simulink model "s0418"  (Simulink 7.0)
settings: Solver=ode3  SolverMode=SingleTasking  StartTime=0.0  StopTime=900  FixedStep=1  MaxStep=1  RelTol=1e-3  AbsTol=1e-6
values from neighbouring files (symbols this model uses):
  Kpr = 10    [m0108d.m]    (also in m0109b.m = 1; m0113c.m; m0404Bsp.m = 3)
  t0A = -1    [m0404Bsp.m]
undefined symbols (not defined in the file or in its folder): edach, T1D, Tn, Tv
settings Model: Creator=froriep  LastModifiedBy=froriep
settings DataIOCC: LimitDataPoints=off  SaveOutput=off  SaveTime=off
settings OptimizationCC: BooleanDataType=off
settings DebuggingCC: SaveWithParameterizedLinksMsg=none  SignalResolutionControl=TryResolveAllWithWarning  SolverPrmCheckMsg=none  MultiTaskDSMMsg=warning  MultiTaskCondExecSysMsg=none  StrictBusMsg=None
settings HardwareCC: TargetUnknown=on
settings RTWCC: IncludeERTFirstTime=on

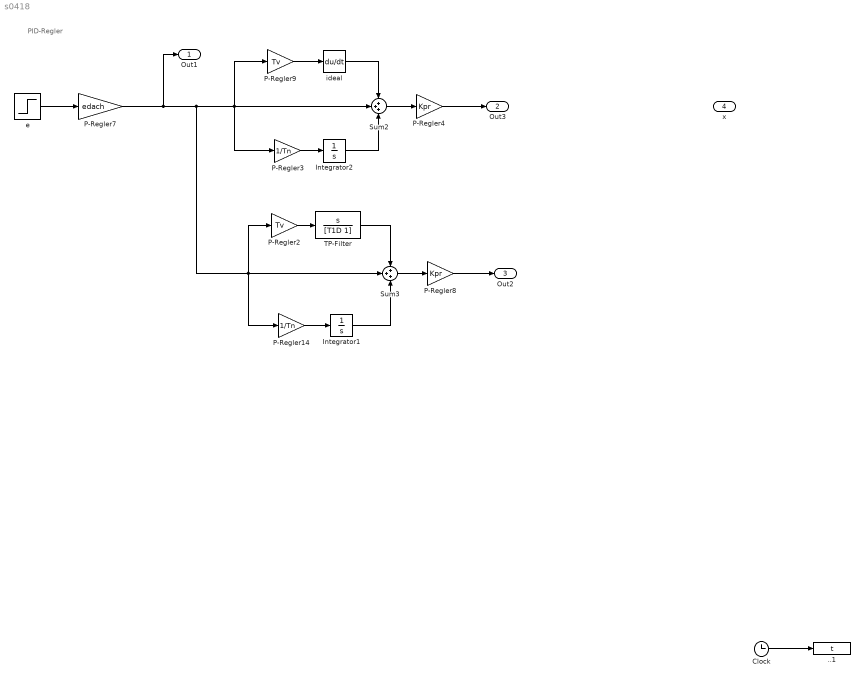
== system s0418 ==
  note: PID-Regler
  ..1 : ToWorkspace  VariableName=t  SaveFormat=Array
  Clock : Clock
      settings: Decimation=10
  Integrator1 : Integrator
  Integrator2 : Integrator
  P-Regler14 : Gain  Gain=1/Tn  ParameterDataType=sfix(16)  ParameterScaling=2^0  OutDataType=sfix(16)  OutScaling=2^0
  P-Regler2 : Gain  Gain=Tv  ParameterDataType=sfix(16)  ParameterScaling=2^0  OutDataType=sfix(16)  OutScaling=2^0
  P-Regler3 : Gain  Gain=1/Tn  ParameterDataType=sfix(16)  ParameterScaling=2^0  OutDataType=sfix(16)  OutScaling=2^0
  P-Regler4 : Gain  Gain=Kpr  ParameterDataType=sfix(16)  ParameterScaling=2^0  OutDataType=sfix(16)  OutScaling=2^0
  P-Regler7 : Gain  Gain=edach  ParameterDataType=sfix(16)  ParameterScaling=2^0  OutDataType=sfix(16)  OutScaling=2^0
  P-Regler8 : Gain  Gain=Kpr  ParameterDataType=sfix(16)  ParameterScaling=2^0  OutDataType=sfix(16)  OutScaling=2^0
  P-Regler9 : Gain  Gain=Tv  ParameterDataType=sfix(16)  ParameterScaling=2^0  OutDataType=sfix(16)  OutScaling=2^0
  Sum2 : Sum  Inputs=+++  SaturateOnIntegerOverflow=on  InputSameDT=on
  Sum3 : Sum  Inputs=+++  SaturateOnIntegerOverflow=on  InputSameDT=on
  TP-Filter : TransferFcn  Numerator=[1 0]  Denominator=[T1D 1]
  e : Step  Time=-t0A  SampleTime=0
  ideal : Derivative
  Out1 : Outport  OutDataType=sfix(16)  OutScaling=2^0
  Out3 : Outport  Port=2  OutDataType=sfix(16)  OutScaling=2^0
  Out2 : Outport  Port=3  OutDataType=sfix(16)  OutScaling=2^0
  x : Outport  Port=4  OutDataType=sfix(16)  OutScaling=2^0
  wires:
  e/1 -> P-Regler7/1
  Clock/1 -> ..1/1
  Sum3/1 -> P-Regler8/1
  P-Regler2/1 -> TP-Filter/1
  TP-Filter/1 -> Sum3/1
  P-Regler7/1 -> Out1/1, P-Regler2/1, Sum3/2, P-Regler14/1, P-Regler9/1, P-Regler3/1, Sum2/2
  P-Regler8/1 -> Out2/1
  P-Regler9/1 -> ideal/1
  ideal/1 -> Sum2/1
  Sum2/1 -> P-Regler4/1
  Integrator1/1 -> Sum3/3
  P-Regler14/1 -> Integrator1/1
  Integrator2/1 -> Sum2/3
  P-Regler3/1 -> Integrator2/1
  P-Regler4/1 -> Out3/1
